simulink library "SIXOSEM_T_STAGE_MONITOR_MASTER"  (Simulink 8.0)
settings: Solver=ode45  StartTime=0.0  StopTime=10.0  RelTol=1e-3
libraries: SIXOSEM_T_MONITOR_MASTER x4
settings Model: Creator=controls  LastModifiedBy=controls

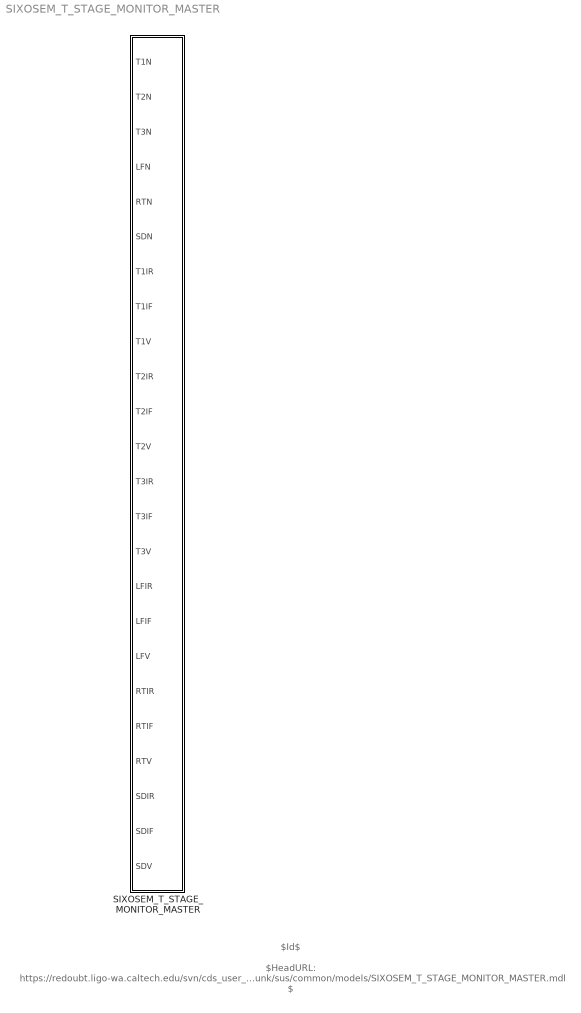
== system SIXOSEM_T_STAGE_MONITOR_MASTER ==
  note: $HeadURL: https://redoubt.ligo-wa.caltech.edu/svn/cds_user_apps/trunk/sus/common/models/SIXOSEM_T_STAGE_MONITOR_MASTER.mdl $
  note: $Id$
  SIXOSEM_T_STAGE_MONITOR_MASTER : Subsystem

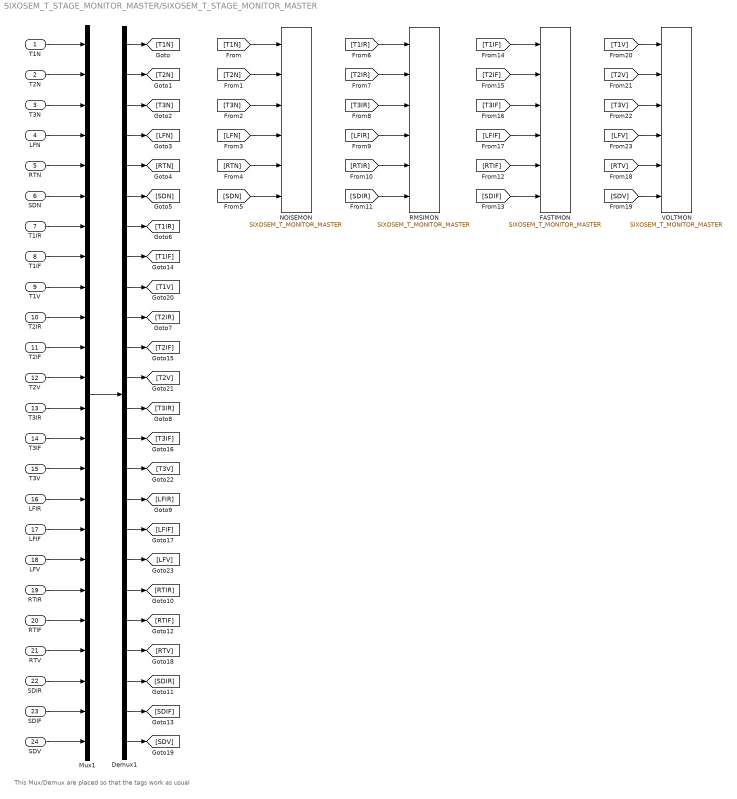
== system SIXOSEM_T_STAGE_MONITOR_MASTER/SIXOSEM_T_STAGE_MONITOR_MASTER ==
  note: This Mux/Demux are placed
      | so that the tags work as usual
  T1N : Inport
  T2N : Inport  Port=2
  T3N : Inport  Port=3
  LFN : Inport  Port=4
  RTN : Inport  Port=5
  SDN : Inport  Port=6
  T1IR : Inport  Port=7
  T1IF : Inport  Port=8
  T1V : Inport  Port=9
  T2IR : Inport  Port=10
  T2IF : Inport  Port=11
  T2V : Inport  Port=12
  T3IR : Inport  Port=13
  T3IF : Inport  Port=14
  T3V : Inport  Port=15
  LFIR : Inport  Port=16
  LFIF : Inport  Port=17
  LFV : Inport  Port=18
  RTIR : Inport  Port=19
  RTIF : Inport  Port=20
  RTV : Inport  Port=21
  SDIR : Inport  Port=22
  SDIF : Inport  Port=23
  SDV : Inport  Port=24
  Demux1 : Demux  Outputs=24
  FASTIMON : SIXOSEM_T_MONITOR_MASTER/SIXOSEM_T_MONITOR_MASTER  SystemSampleTime=-1
  Mux1 : Mux  Inputs=24
  NOISEMON : SIXOSEM_T_MONITOR_MASTER/SIXOSEM_T_MONITOR_MASTER  SystemSampleTime=-1
  RMSIMON : SIXOSEM_T_MONITOR_MASTER/SIXOSEM_T_MONITOR_MASTER  SystemSampleTime=-1
  VOLTMON : SIXOSEM_T_MONITOR_MASTER/SIXOSEM_T_MONITOR_MASTER  SystemSampleTime=-1
  wires:
  T1N/1 -> Mux1/1
  SDV/1 -> Mux1/24
  SDIF/1 -> Mux1/23
  SDIR/1 -> Mux1/22
  T2V/1 -> Mux1/12
  T3IR/1 -> Mux1/13
  T3IF/1 -> Mux1/14
  T3V/1 -> Mux1/15
  LFIR/1 -> Mux1/16
  LFIF/1 -> Mux1/17
  LFV/1 -> Mux1/18
  RTIR/1 -> Mux1/19
  RTIF/1 -> Mux1/20
  RTV/1 -> Mux1/21
  T2N/1 -> Mux1/2
  T3N/1 -> Mux1/3
  LFN/1 -> Mux1/4
  RTN/1 -> Mux1/5
  SDN/1 -> Mux1/6
  T1IR/1 -> Mux1/7
  T1IF/1 -> Mux1/8
  T1V/1 -> Mux1/9
  T2IR/1 -> Mux1/10
  T2IF/1 -> Mux1/11
  Mux1/1 -> Demux1/1
  [T1N] -> NOISEMON/1
  Demux1/1 -> [T1N]
  Demux1/2 -> [T2N]
  Demux1/3 -> [T3N]
  Demux1/4 -> [LFN]
  Demux1/5 -> [RTN]
  Demux1/6 -> [SDN]
  [T2N] -> NOISEMON/2
  [T3N] -> NOISEMON/3
  [RTN] -> NOISEMON/5
  [SDN] -> NOISEMON/6
  [LFN] -> NOISEMON/4
  [T1IR] -> RMSIMON/1
  [T2IR] -> RMSIMON/2
  [T3IR] -> RMSIMON/3
  [RTIR] -> RMSIMON/5
  [SDIR] -> RMSIMON/6
  [LFIR] -> RMSIMON/4
  Demux1/7 -> [T1IR]
  Demux1/8 -> [T1IF]
  Demux1/9 -> [T1V]
  Demux1/10 -> [T2IR]
  Demux1/11 -> [T2IF]
  Demux1/12 -> [T2V]
  Demux1/13 -> [T3IR]
  Demux1/14 -> [T3IF]
  Demux1/15 -> [T3V]
  Demux1/16 -> [LFIR]
  Demux1/17 -> [LFIF]
  Demux1/18 -> [LFV]
  Demux1/19 -> [RTIR]
  Demux1/20 -> [RTIF]
  Demux1/21 -> [RTV]
  Demux1/22 -> [SDIR]
  Demux1/23 -> [SDIF]
  Demux1/24 -> [SDV]
  [T1IF] -> FASTIMON/1
  [T2IF] -> FASTIMON/2
  [T3IF] -> FASTIMON/3
  [RTIF] -> FASTIMON/5
  [SDIF] -> FASTIMON/6
  [LFIF] -> FASTIMON/4
  [T1V] -> VOLTMON/1
  [T2V] -> VOLTMON/2
  [T3V] -> VOLTMON/3
  [RTV] -> VOLTMON/5
  [SDV] -> VOLTMON/6
  [LFV] -> VOLTMON/4
